simulink model "Subsystem0"  (R2020a)
settings: Solver=VariableStepAuto  StartTime=0.0  StopTime=120  RelTol=1e-3
undefined symbols (not defined in the file or in its folder): D, I, P
settings Model: DataDictionary=ModelData.sldd  Creator=tnradm  LastModifiedBy=tnradm
settings DataIOCC: SaveOutput=off  SaveTime=off

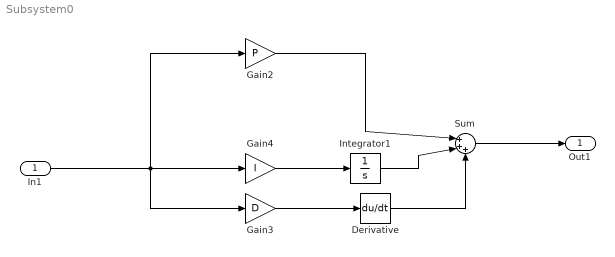
== system Subsystem0 ==
  In1 : Inport  OutDataTypeStr=double  PortDimensions=1  SampleTime=0
  Derivative : Derivative
  Gain2 : Gain  Gain=P
  Gain3 : Gain  Gain=D
  Gain4 : Gain  Gain=I
  Integrator1 : Integrator
  Sum : Sum  Inputs=|+++
  Out1 : Outport  OutDataTypeStr=double  PortDimensions=1  SampleTime=0
  wires:
  Sum/1 -> Out1/1
  Gain3/1 -> Derivative/1
  In1/1 -> Gain4/1, Gain3/1, Gain2/1
  Derivative/1 -> Sum/3
  Gain4/1 -> Integrator1/1
  Integrator1/1 -> Sum/2
  Gain2/1 -> Sum/1
